simulink model "tracker"  (R2020a)
settings: Solver=VariableStepAuto  StartTime=0.0  StopTime=simulation_time  RelTol=1e-3
values from neighbouring files (symbols this model uses):
  costas_pll_arctan_nstage = 8    [tracker_hw_init.m]
  costas_pll_arctan_point = 16    [tracker_hw_init.m]
  costas_pll_arctan_width = 32    [tracker_hw_init.m]
  DDS_ch_pinc = fc.*(2^(DDS_phase_width)/fs)    [tracker_hw_init.m]
  fs = 120e6    (= 120000000)    [tracker_hw_init.m]
  normalized_EML_power_cordic_nstage = 11    [tracker_hw_init.m]
  normalized_EML_power_cordic_point = 32    [tracker_hw_init.m]
  normalized_EML_power_cordic_width = 32    [tracker_hw_init.m]
  ts = 1/fs    (= 8.33333333333e-09)    [tracker_hw_init.m]
undefined symbols (not defined in the file or in its folder): cacode, i
libraries: xbsIndex_r4 x1873
(part 3 of 14)

== system tracker/CA_code_bank/input_router/address_router1 ==
  ca_select : Inport
  Mux{,1..10} (11 alike) : xbsIndex_r4/Mux  inputs=2  en=off  latency=1  precision=Full  arith_type=Unsigned  n_bits=16  bin_pt=14  quantization=Truncate  overflow=Wrap  dbl_ovrd=off  block_type=mux
  Relational{,1..10} (11 alike) : xbsIndex_r4/Relational  mode=a=b  op_type=Bool  en=off  latency=1  dbl_ovrd=off  block_type=relational
  ca_addr : Outport
  wires:
  [CA_code_addr_ch11] -> Mux10/3
  Mux8/1 -> Mux7/2
  Mux5/1 -> Mux4/2
  [CA_code_select_ch8] -> Relational7/1
  [CA_code_addr_ch9] -> Mux8/3
  [CA_code_select_ch7] -> Relational6/1
  Relational/1 -> Mux/1
  [CA_code_addr_ch1] -> Mux/3
  Mux9/1 -> Mux8/2
  ca_select/1 -> Relational1/2, Relational2/2, Relational3/2, Relational4/2, Relational5/2, Relational6/2, Relational7/2, Relational8/2, Relational9/2, Relational10/2, Relational/2
  Relational9/1 -> Mux9/1
  Mux3/1 -> Mux2/2
  [CA_code_select_ch4] -> Relational3/1
  [CA_code_select_ch3] -> Relational2/1
  Relational8/1 -> Mux8/1
  Relational2/1 -> Mux2/1
  [CA_code_addr_ch5] -> Mux4/3
  [CA_code_select_ch5] -> Relational4/1
  Relational10/1 -> Mux10/1
  Mux2/1 -> Mux1/2
  [CA_code_select_ch2] -> Relational1/1
  Mux4/1 -> Mux3/2
  Relational7/1 -> Mux7/1
  Relational4/1 -> Mux4/1
  [CA_code_select_ch6] -> Relational5/1
  [CA_code_addr_ch6] -> Mux5/3
  [CA_code_addr_ch3] -> Mux2/3
  [CA_code_select_ch1] -> Relational/1
  [CA_code_addr_ch4] -> Mux3/3
  Relational3/1 -> Mux3/1
  [CA_code_select_ch11] -> Relational10/1
  [CA_code_select_ch10] -> Relational9/1
  [CA_code_select_ch9] -> Relational8/1
  Relational5/1 -> Mux5/1
  Mux10/1 -> Mux9/2
  [CA_code_addr_ch10] -> Mux9/3
  Mux7/1 -> Mux6/2
  [CA_code_addr_ch12] -> Mux10/2
  Relational1/1 -> Mux1/1
  [CA_code_addr_ch8] -> Mux7/3
  [CA_code_addr_ch7] -> Mux6/3
  Mux1/1 -> Mux/2
  [CA_code_addr_ch2] -> Mux1/3
  Relational6/1 -> Mux6/1
  Mux6/1 -> Mux5/2
  Mux/1 -> ca_addr/1

== system tracker/CA_code_bank/input_router/address_router10 ==
  ca_select : Inport
  Mux{,1..10} (11 alike) : xbsIndex_r4/Mux  inputs=2  en=off  latency=1  precision=Full  arith_type=Unsigned  n_bits=16  bin_pt=14  quantization=Truncate  overflow=Wrap  dbl_ovrd=off  block_type=mux
  Relational{,1..10} (11 alike) : xbsIndex_r4/Relational  mode=a=b  op_type=Bool  en=off  latency=1  dbl_ovrd=off  block_type=relational
  ca_addr : Outport
  wires:
  [CA_code_addr_ch11] -> Mux10/3
  Mux8/1 -> Mux7/2
  Mux5/1 -> Mux4/2
  [CA_code_select_ch8] -> Relational7/1
  [CA_code_addr_ch9] -> Mux8/3
  [CA_code_select_ch7] -> Relational6/1
  Relational/1 -> Mux/1
  [CA_code_addr_ch1] -> Mux/3
  Mux9/1 -> Mux8/2
  ca_select/1 -> Relational1/2, Relational2/2, Relational3/2, Relational4/2, Relational5/2, Relational6/2, Relational7/2, Relational8/2, Relational9/2, Relational10/2, Relational/2
  Relational9/1 -> Mux9/1
  Mux3/1 -> Mux2/2
  [CA_code_select_ch4] -> Relational3/1
  [CA_code_select_ch3] -> Relational2/1
  Relational8/1 -> Mux8/1
  Relational2/1 -> Mux2/1
  [CA_code_addr_ch5] -> Mux4/3
  [CA_code_select_ch5] -> Relational4/1
  Relational10/1 -> Mux10/1
  Mux2/1 -> Mux1/2
  [CA_code_select_ch2] -> Relational1/1
  Mux4/1 -> Mux3/2
  Relational7/1 -> Mux7/1
  Relational4/1 -> Mux4/1
  [CA_code_select_ch6] -> Relational5/1
  [CA_code_addr_ch6] -> Mux5/3
  [CA_code_addr_ch3] -> Mux2/3
  [CA_code_select_ch1] -> Relational/1
  [CA_code_addr_ch4] -> Mux3/3
  Relational3/1 -> Mux3/1
  [CA_code_select_ch11] -> Relational10/1
  [CA_code_select_ch10] -> Relational9/1
  [CA_code_select_ch9] -> Relational8/1
  Relational5/1 -> Mux5/1
  Mux10/1 -> Mux9/2
  [CA_code_addr_ch10] -> Mux9/3
  Mux7/1 -> Mux6/2
  [CA_code_addr_ch12] -> Mux10/2
  Relational1/1 -> Mux1/1
  [CA_code_addr_ch8] -> Mux7/3
  [CA_code_addr_ch7] -> Mux6/3
  Mux1/1 -> Mux/2
  [CA_code_addr_ch2] -> Mux1/3
  Relational6/1 -> Mux6/1
  Mux6/1 -> Mux5/2
  Mux/1 -> ca_addr/1

== system tracker/CA_code_bank/input_router/address_router11 ==
  ca_select : Inport
  Mux{,1..10} (11 alike) : xbsIndex_r4/Mux  inputs=2  en=off  latency=1  precision=Full  arith_type=Unsigned  n_bits=16  bin_pt=14  quantization=Truncate  overflow=Wrap  dbl_ovrd=off  block_type=mux
  Relational{,1..10} (11 alike) : xbsIndex_r4/Relational  mode=a=b  op_type=Bool  en=off  latency=1  dbl_ovrd=off  block_type=relational
  ca_addr : Outport
  wires:
  Mux/1 -> ca_addr/1
  Mux6/1 -> Mux5/2
  Relational6/1 -> Mux6/1
  [CA_code_addr_ch2] -> Mux1/3
  Mux1/1 -> Mux/2
  [CA_code_addr_ch7] -> Mux6/3
  [CA_code_addr_ch8] -> Mux7/3
  Relational1/1 -> Mux1/1
  [CA_code_addr_ch12] -> Mux10/2
  Mux7/1 -> Mux6/2
  [CA_code_addr_ch10] -> Mux9/3
  Mux10/1 -> Mux9/2
  Relational5/1 -> Mux5/1
  [CA_code_select_ch9] -> Relational8/1
  [CA_code_select_ch10] -> Relational9/1
  [CA_code_select_ch11] -> Relational10/1
  Relational3/1 -> Mux3/1
  [CA_code_addr_ch4] -> Mux3/3
  [CA_code_select_ch1] -> Relational/1
  [CA_code_addr_ch3] -> Mux2/3
  [CA_code_addr_ch6] -> Mux5/3
  [CA_code_select_ch6] -> Relational5/1
  Relational4/1 -> Mux4/1
  Relational7/1 -> Mux7/1
  Mux4/1 -> Mux3/2
  [CA_code_select_ch2] -> Relational1/1
  Mux2/1 -> Mux1/2
  Relational10/1 -> Mux10/1
  [CA_code_select_ch5] -> Relational4/1
  [CA_code_addr_ch5] -> Mux4/3
  Relational2/1 -> Mux2/1
  Relational8/1 -> Mux8/1
  [CA_code_select_ch3] -> Relational2/1
  [CA_code_select_ch4] -> Relational3/1
  Mux3/1 -> Mux2/2
  Relational9/1 -> Mux9/1
  ca_select/1 -> Relational/2, Relational10/2, Relational9/2, Relational8/2, Relational7/2, Relational6/2, Relational5/2, Relational4/2, Relational3/2, Relational2/2, Relational1/2
  Mux9/1 -> Mux8/2
  [CA_code_addr_ch1] -> Mux/3
  Relational/1 -> Mux/1
  [CA_code_select_ch7] -> Relational6/1
  [CA_code_addr_ch9] -> Mux8/3
  [CA_code_select_ch8] -> Relational7/1
  Mux5/1 -> Mux4/2
  Mux8/1 -> Mux7/2
  [CA_code_addr_ch11] -> Mux10/3

== system tracker/CA_code_bank/input_router/address_router12 ==
  ca_select : Inport
  Mux{,1..10} (11 alike) : xbsIndex_r4/Mux  inputs=2  en=off  latency=1  precision=Full  arith_type=Unsigned  n_bits=16  bin_pt=14  quantization=Truncate  overflow=Wrap  dbl_ovrd=off  block_type=mux
  Relational{,1..10} (11 alike) : xbsIndex_r4/Relational  mode=a=b  op_type=Bool  en=off  latency=1  dbl_ovrd=off  block_type=relational
  ca_addr : Outport
  wires:
  [CA_code_addr_ch11] -> Mux10/3
  Mux8/1 -> Mux7/2
  Mux5/1 -> Mux4/2
  [CA_code_select_ch8] -> Relational7/1
  [CA_code_addr_ch9] -> Mux8/3
  [CA_code_select_ch7] -> Relational6/1
  Relational/1 -> Mux/1
  [CA_code_addr_ch1] -> Mux/3
  Mux9/1 -> Mux8/2
  ca_select/1 -> Relational1/2, Relational2/2, Relational3/2, Relational4/2, Relational5/2, Relational6/2, Relational7/2, Relational8/2, Relational9/2, Relational10/2, Relational/2
  Relational9/1 -> Mux9/1
  Mux3/1 -> Mux2/2
  [CA_code_select_ch4] -> Relational3/1
  [CA_code_select_ch3] -> Relational2/1
  Relational8/1 -> Mux8/1
  Relational2/1 -> Mux2/1
  [CA_code_addr_ch5] -> Mux4/3
  [CA_code_select_ch5] -> Relational4/1
  Relational10/1 -> Mux10/1
  Mux2/1 -> Mux1/2
  [CA_code_select_ch2] -> Relational1/1
  Mux4/1 -> Mux3/2
  Relational7/1 -> Mux7/1
  Relational4/1 -> Mux4/1
  [CA_code_select_ch6] -> Relational5/1
  [CA_code_addr_ch6] -> Mux5/3
  [CA_code_addr_ch3] -> Mux2/3
  [CA_code_select_ch1] -> Relational/1
  [CA_code_addr_ch4] -> Mux3/3
  Relational3/1 -> Mux3/1
  [CA_code_select_ch11] -> Relational10/1
  [CA_code_select_ch10] -> Relational9/1
  [CA_code_select_ch9] -> Relational8/1
  Relational5/1 -> Mux5/1
  Mux10/1 -> Mux9/2
  [CA_code_addr_ch10] -> Mux9/3
  Mux7/1 -> Mux6/2
  [CA_code_addr_ch12] -> Mux10/2
  Relational1/1 -> Mux1/1
  [CA_code_addr_ch8] -> Mux7/3
  [CA_code_addr_ch7] -> Mux6/3
  Mux1/1 -> Mux/2
  [CA_code_addr_ch2] -> Mux1/3
  Relational6/1 -> Mux6/1
  Mux6/1 -> Mux5/2
  Mux/1 -> ca_addr/1

== system tracker/CA_code_bank/input_router/address_router13 ==
  ca_select : Inport
  Mux{,1..10} (11 alike) : xbsIndex_r4/Mux  inputs=2  en=off  latency=1  precision=Full  arith_type=Unsigned  n_bits=16  bin_pt=14  quantization=Truncate  overflow=Wrap  dbl_ovrd=off  block_type=mux
  Relational{,1..10} (11 alike) : xbsIndex_r4/Relational  mode=a=b  op_type=Bool  en=off  latency=1  dbl_ovrd=off  block_type=relational
  ca_addr : Outport
  wires:
  Mux/1 -> ca_addr/1
  Mux6/1 -> Mux5/2
  Relational6/1 -> Mux6/1
  [CA_code_addr_ch2] -> Mux1/3
  Mux1/1 -> Mux/2
  [CA_code_addr_ch7] -> Mux6/3
  [CA_code_addr_ch8] -> Mux7/3
  Relational1/1 -> Mux1/1
  [CA_code_addr_ch12] -> Mux10/2
  Mux7/1 -> Mux6/2
  [CA_code_addr_ch10] -> Mux9/3
  Mux10/1 -> Mux9/2
  Relational5/1 -> Mux5/1
  [CA_code_select_ch9] -> Relational8/1
  [CA_code_select_ch10] -> Relational9/1
  [CA_code_select_ch11] -> Relational10/1
  Relational3/1 -> Mux3/1
  [CA_code_addr_ch4] -> Mux3/3
  [CA_code_select_ch1] -> Relational/1
  [CA_code_addr_ch3] -> Mux2/3
  [CA_code_addr_ch6] -> Mux5/3
  [CA_code_select_ch6] -> Relational5/1
  Relational4/1 -> Mux4/1
  Relational7/1 -> Mux7/1
  Mux4/1 -> Mux3/2
  [CA_code_select_ch2] -> Relational1/1
  Mux2/1 -> Mux1/2
  Relational10/1 -> Mux10/1
  [CA_code_select_ch5] -> Relational4/1
  [CA_code_addr_ch5] -> Mux4/3
  Relational2/1 -> Mux2/1
  Relational8/1 -> Mux8/1
  [CA_code_select_ch3] -> Relational2/1
  [CA_code_select_ch4] -> Relational3/1
  Mux3/1 -> Mux2/2
  Relational9/1 -> Mux9/1
  ca_select/1 -> Relational/2, Relational10/2, Relational9/2, Relational8/2, Relational7/2, Relational6/2, Relational5/2, Relational4/2, Relational3/2, Relational2/2, Relational1/2
  Mux9/1 -> Mux8/2
  [CA_code_addr_ch1] -> Mux/3
  Relational/1 -> Mux/1
  [CA_code_select_ch7] -> Relational6/1
  [CA_code_addr_ch9] -> Mux8/3
  [CA_code_select_ch8] -> Relational7/1
  Mux5/1 -> Mux4/2
  Mux8/1 -> Mux7/2
  [CA_code_addr_ch11] -> Mux10/3

== system tracker/CA_code_bank/input_router/address_router14 ==
  ca_select : Inport
  Mux{,1..10} (11 alike) : xbsIndex_r4/Mux  inputs=2  en=off  latency=1  precision=Full  arith_type=Unsigned  n_bits=16  bin_pt=14  quantization=Truncate  overflow=Wrap  dbl_ovrd=off  block_type=mux
  Relational{,1..10} (11 alike) : xbsIndex_r4/Relational  mode=a=b  op_type=Bool  en=off  latency=1  dbl_ovrd=off  block_type=relational
  ca_addr : Outport
  wires:
  Mux/1 -> ca_addr/1
  Mux6/1 -> Mux5/2
  Relational6/1 -> Mux6/1
  [CA_code_addr_ch2] -> Mux1/3
  Mux1/1 -> Mux/2
  [CA_code_addr_ch7] -> Mux6/3
  [CA_code_addr_ch8] -> Mux7/3
  Relational1/1 -> Mux1/1
  [CA_code_addr_ch12] -> Mux10/2
  Mux7/1 -> Mux6/2
  [CA_code_addr_ch10] -> Mux9/3
  Mux10/1 -> Mux9/2
  Relational5/1 -> Mux5/1
  [CA_code_select_ch9] -> Relational8/1
  [CA_code_select_ch10] -> Relational9/1
  [CA_code_select_ch11] -> Relational10/1
  Relational3/1 -> Mux3/1
  [CA_code_addr_ch4] -> Mux3/3
  [CA_code_select_ch1] -> Relational/1
  [CA_code_addr_ch3] -> Mux2/3
  [CA_code_addr_ch6] -> Mux5/3
  [CA_code_select_ch6] -> Relational5/1
  Relational4/1 -> Mux4/1
  Relational7/1 -> Mux7/1
  Mux4/1 -> Mux3/2
  [CA_code_select_ch2] -> Relational1/1
  Mux2/1 -> Mux1/2
  Relational10/1 -> Mux10/1
  [CA_code_select_ch5] -> Relational4/1
  [CA_code_addr_ch5] -> Mux4/3
  Relational2/1 -> Mux2/1
  Relational8/1 -> Mux8/1
  [CA_code_select_ch3] -> Relational2/1
  [CA_code_select_ch4] -> Relational3/1
  Mux3/1 -> Mux2/2
  Relational9/1 -> Mux9/1
  ca_select/1 -> Relational/2, Relational10/2, Relational9/2, Relational8/2, Relational7/2, Relational6/2, Relational5/2, Relational4/2, Relational3/2, Relational2/2, Relational1/2
  Mux9/1 -> Mux8/2
  [CA_code_addr_ch1] -> Mux/3
  Relational/1 -> Mux/1
  [CA_code_select_ch7] -> Relational6/1
  [CA_code_addr_ch9] -> Mux8/3
  [CA_code_select_ch8] -> Relational7/1
  Mux5/1 -> Mux4/2
  Mux8/1 -> Mux7/2
  [CA_code_addr_ch11] -> Mux10/3

== system tracker/CA_code_bank/input_router/address_router15 ==
  ca_select : Inport
  Mux{,1..10} (11 alike) : xbsIndex_r4/Mux  inputs=2  en=off  latency=1  precision=Full  arith_type=Unsigned  n_bits=16  bin_pt=14  quantization=Truncate  overflow=Wrap  dbl_ovrd=off  block_type=mux
  Relational{,1..10} (11 alike) : xbsIndex_r4/Relational  mode=a=b  op_type=Bool  en=off  latency=1  dbl_ovrd=off  block_type=relational
  ca_addr : Outport
  wires:
  [CA_code_addr_ch11] -> Mux10/3
  Mux8/1 -> Mux7/2
  Mux5/1 -> Mux4/2
  [CA_code_select_ch8] -> Relational7/1
  [CA_code_addr_ch9] -> Mux8/3
  [CA_code_select_ch7] -> Relational6/1
  Relational/1 -> Mux/1
  [CA_code_addr_ch1] -> Mux/3
  Mux9/1 -> Mux8/2
  ca_select/1 -> Relational1/2, Relational2/2, Relational3/2, Relational4/2, Relational5/2, Relational6/2, Relational7/2, Relational8/2, Relational9/2, Relational10/2, Relational/2
  Relational9/1 -> Mux9/1
  Mux3/1 -> Mux2/2
  [CA_code_select_ch4] -> Relational3/1
  [CA_code_select_ch3] -> Relational2/1
  Relational8/1 -> Mux8/1
  Relational2/1 -> Mux2/1
  [CA_code_addr_ch5] -> Mux4/3
  [CA_code_select_ch5] -> Relational4/1
  Relational10/1 -> Mux10/1
  Mux2/1 -> Mux1/2
  [CA_code_select_ch2] -> Relational1/1
  Mux4/1 -> Mux3/2
  Relational7/1 -> Mux7/1
  Relational4/1 -> Mux4/1
  [CA_code_select_ch6] -> Relational5/1
  [CA_code_addr_ch6] -> Mux5/3
  [CA_code_addr_ch3] -> Mux2/3
  [CA_code_select_ch1] -> Relational/1
  [CA_code_addr_ch4] -> Mux3/3
  Relational3/1 -> Mux3/1
  [CA_code_select_ch11] -> Relational10/1
  [CA_code_select_ch10] -> Relational9/1
  [CA_code_select_ch9] -> Relational8/1
  Relational5/1 -> Mux5/1
  Mux10/1 -> Mux9/2
  [CA_code_addr_ch10] -> Mux9/3
  Mux7/1 -> Mux6/2
  [CA_code_addr_ch12] -> Mux10/2
  Relational1/1 -> Mux1/1
  [CA_code_addr_ch8] -> Mux7/3
  [CA_code_addr_ch7] -> Mux6/3
  Mux1/1 -> Mux/2
  [CA_code_addr_ch2] -> Mux1/3
  Relational6/1 -> Mux6/1
  Mux6/1 -> Mux5/2
  Mux/1 -> ca_addr/1

== system tracker/CA_code_bank/input_router/address_router16 ==
  ca_select : Inport
  Mux{,1..10} (11 alike) : xbsIndex_r4/Mux  inputs=2  en=off  latency=1  precision=Full  arith_type=Unsigned  n_bits=16  bin_pt=14  quantization=Truncate  overflow=Wrap  dbl_ovrd=off  block_type=mux
  Relational{,1..10} (11 alike) : xbsIndex_r4/Relational  mode=a=b  op_type=Bool  en=off  latency=1  dbl_ovrd=off  block_type=relational
  ca_addr : Outport
  wires:
  Mux/1 -> ca_addr/1
  Mux6/1 -> Mux5/2
  Relational6/1 -> Mux6/1
  [CA_code_addr_ch2] -> Mux1/3
  Mux1/1 -> Mux/2
  [CA_code_addr_ch7] -> Mux6/3
  [CA_code_addr_ch8] -> Mux7/3
  Relational1/1 -> Mux1/1
  [CA_code_addr_ch12] -> Mux10/2
  Mux7/1 -> Mux6/2
  [CA_code_addr_ch10] -> Mux9/3
  Mux10/1 -> Mux9/2
  Relational5/1 -> Mux5/1
  [CA_code_select_ch9] -> Relational8/1
  [CA_code_select_ch10] -> Relational9/1
  [CA_code_select_ch11] -> Relational10/1
  Relational3/1 -> Mux3/1
  [CA_code_addr_ch4] -> Mux3/3
  [CA_code_select_ch1] -> Relational/1
  [CA_code_addr_ch3] -> Mux2/3
  [CA_code_addr_ch6] -> Mux5/3
  [CA_code_select_ch6] -> Relational5/1
  Relational4/1 -> Mux4/1
  Relational7/1 -> Mux7/1
  Mux4/1 -> Mux3/2
  [CA_code_select_ch2] -> Relational1/1
  Mux2/1 -> Mux1/2
  Relational10/1 -> Mux10/1
  [CA_code_select_ch5] -> Relational4/1
  [CA_code_addr_ch5] -> Mux4/3
  Relational2/1 -> Mux2/1
  Relational8/1 -> Mux8/1
  [CA_code_select_ch3] -> Relational2/1
  [CA_code_select_ch4] -> Relational3/1
  Mux3/1 -> Mux2/2
  Relational9/1 -> Mux9/1
  ca_select/1 -> Relational/2, Relational10/2, Relational9/2, Relational8/2, Relational7/2, Relational6/2, Relational5/2, Relational4/2, Relational3/2, Relational2/2, Relational1/2
  Mux9/1 -> Mux8/2
  [CA_code_addr_ch1] -> Mux/3
  Relational/1 -> Mux/1
  [CA_code_select_ch7] -> Relational6/1
  [CA_code_addr_ch9] -> Mux8/3
  [CA_code_select_ch8] -> Relational7/1
  Mux5/1 -> Mux4/2
  Mux8/1 -> Mux7/2
  [CA_code_addr_ch11] -> Mux10/3

== system tracker/CA_code_bank/input_router/address_router17 ==
  ca_select : Inport
  Mux{,1..10} (11 alike) : xbsIndex_r4/Mux  inputs=2  en=off  latency=1  precision=Full  arith_type=Unsigned  n_bits=16  bin_pt=14  quantization=Truncate  overflow=Wrap  dbl_ovrd=off  block_type=mux
  Relational{,1..10} (11 alike) : xbsIndex_r4/Relational  mode=a=b  op_type=Bool  en=off  latency=1  dbl_ovrd=off  block_type=relational
  ca_addr : Outport
  wires:
  [CA_code_addr_ch11] -> Mux10/3
  Mux8/1 -> Mux7/2
  Mux5/1 -> Mux4/2
  [CA_code_select_ch8] -> Relational7/1
  [CA_code_addr_ch9] -> Mux8/3
  [CA_code_select_ch7] -> Relational6/1
  Relational/1 -> Mux/1
  [CA_code_addr_ch1] -> Mux/3
  Mux9/1 -> Mux8/2
  ca_select/1 -> Relational1/2, Relational2/2, Relational3/2, Relational4/2, Relational5/2, Relational6/2, Relational7/2, Relational8/2, Relational9/2, Relational10/2, Relational/2
  Relational9/1 -> Mux9/1
  Mux3/1 -> Mux2/2
  [CA_code_select_ch4] -> Relational3/1
  [CA_code_select_ch3] -> Relational2/1
  Relational8/1 -> Mux8/1
  Relational2/1 -> Mux2/1
  [CA_code_addr_ch5] -> Mux4/3
  [CA_code_select_ch5] -> Relational4/1
  Relational10/1 -> Mux10/1
  Mux2/1 -> Mux1/2
  [CA_code_select_ch2] -> Relational1/1
  Mux4/1 -> Mux3/2
  Relational7/1 -> Mux7/1
  Relational4/1 -> Mux4/1
  [CA_code_select_ch6] -> Relational5/1
  [CA_code_addr_ch6] -> Mux5/3
  [CA_code_addr_ch3] -> Mux2/3
  [CA_code_select_ch1] -> Relational/1
  [CA_code_addr_ch4] -> Mux3/3
  Relational3/1 -> Mux3/1
  [CA_code_select_ch11] -> Relational10/1
  [CA_code_select_ch10] -> Relational9/1
  [CA_code_select_ch9] -> Relational8/1
  Relational5/1 -> Mux5/1
  Mux10/1 -> Mux9/2
  [CA_code_addr_ch10] -> Mux9/3
  Mux7/1 -> Mux6/2
  [CA_code_addr_ch12] -> Mux10/2
  Relational1/1 -> Mux1/1
  [CA_code_addr_ch8] -> Mux7/3
  [CA_code_addr_ch7] -> Mux6/3
  Mux1/1 -> Mux/2
  [CA_code_addr_ch2] -> Mux1/3
  Relational6/1 -> Mux6/1
  Mux6/1 -> Mux5/2
  Mux/1 -> ca_addr/1

== system tracker/CA_code_bank/input_router/address_router18 ==
  ca_select : Inport
  Mux{,1..10} (11 alike) : xbsIndex_r4/Mux  inputs=2  en=off  latency=1  precision=Full  arith_type=Unsigned  n_bits=16  bin_pt=14  quantization=Truncate  overflow=Wrap  dbl_ovrd=off  block_type=mux
  Relational{,1..10} (11 alike) : xbsIndex_r4/Relational  mode=a=b  op_type=Bool  en=off  latency=1  dbl_ovrd=off  block_type=relational
  ca_addr : Outport
  wires:
  Mux/1 -> ca_addr/1
  Mux6/1 -> Mux5/2
  Relational6/1 -> Mux6/1
  [CA_code_addr_ch2] -> Mux1/3
  Mux1/1 -> Mux/2
  [CA_code_addr_ch7] -> Mux6/3
  [CA_code_addr_ch8] -> Mux7/3
  Relational1/1 -> Mux1/1
  [CA_code_addr_ch12] -> Mux10/2
  Mux7/1 -> Mux6/2
  [CA_code_addr_ch10] -> Mux9/3
  Mux10/1 -> Mux9/2
  Relational5/1 -> Mux5/1
  [CA_code_select_ch9] -> Relational8/1
  [CA_code_select_ch10] -> Relational9/1
  [CA_code_select_ch11] -> Relational10/1
  Relational3/1 -> Mux3/1
  [CA_code_addr_ch4] -> Mux3/3
  [CA_code_select_ch1] -> Relational/1
  [CA_code_addr_ch3] -> Mux2/3
  [CA_code_addr_ch6] -> Mux5/3
  [CA_code_select_ch6] -> Relational5/1
  Relational4/1 -> Mux4/1
  Relational7/1 -> Mux7/1
  Mux4/1 -> Mux3/2
  [CA_code_select_ch2] -> Relational1/1
  Mux2/1 -> Mux1/2
  Relational10/1 -> Mux10/1
  [CA_code_select_ch5] -> Relational4/1
  [CA_code_addr_ch5] -> Mux4/3
  Relational2/1 -> Mux2/1
  Relational8/1 -> Mux8/1
  [CA_code_select_ch3] -> Relational2/1
  [CA_code_select_ch4] -> Relational3/1
  Mux3/1 -> Mux2/2
  Relational9/1 -> Mux9/1
  ca_select/1 -> Relational/2, Relational10/2, Relational9/2, Relational8/2, Relational7/2, Relational6/2, Relational5/2, Relational4/2, Relational3/2, Relational2/2, Relational1/2
  Mux9/1 -> Mux8/2
  [CA_code_addr_ch1] -> Mux/3
  Relational/1 -> Mux/1
  [CA_code_select_ch7] -> Relational6/1
  [CA_code_addr_ch9] -> Mux8/3
  [CA_code_select_ch8] -> Relational7/1
  Mux5/1 -> Mux4/2
  Mux8/1 -> Mux7/2
  [CA_code_addr_ch11] -> Mux10/3

== system tracker/CA_code_bank/input_router/address_router19 ==
  ca_select : Inport
  Mux{,1..10} (11 alike) : xbsIndex_r4/Mux  inputs=2  en=off  latency=1  precision=Full  arith_type=Unsigned  n_bits=16  bin_pt=14  quantization=Truncate  overflow=Wrap  dbl_ovrd=off  block_type=mux
  Relational{,1..10} (11 alike) : xbsIndex_r4/Relational  mode=a=b  op_type=Bool  en=off  latency=1  dbl_ovrd=off  block_type=relational
  ca_addr : Outport
  wires:
  [CA_code_addr_ch11] -> Mux10/3
  Mux8/1 -> Mux7/2
  Mux5/1 -> Mux4/2
  [CA_code_select_ch8] -> Relational7/1
  [CA_code_addr_ch9] -> Mux8/3
  [CA_code_select_ch7] -> Relational6/1
  Relational/1 -> Mux/1
  [CA_code_addr_ch1] -> Mux/3
  Mux9/1 -> Mux8/2
  ca_select/1 -> Relational1/2, Relational2/2, Relational3/2, Relational4/2, Relational5/2, Relational6/2, Relational7/2, Relational8/2, Relational9/2, Relational10/2, Relational/2
  Relational9/1 -> Mux9/1
  Mux3/1 -> Mux2/2
  [CA_code_select_ch4] -> Relational3/1
  [CA_code_select_ch3] -> Relational2/1
  Relational8/1 -> Mux8/1
  Relational2/1 -> Mux2/1
  [CA_code_addr_ch5] -> Mux4/3
  [CA_code_select_ch5] -> Relational4/1
  Relational10/1 -> Mux10/1
  Mux2/1 -> Mux1/2
  [CA_code_select_ch2] -> Relational1/1
  Mux4/1 -> Mux3/2
  Relational7/1 -> Mux7/1
  Relational4/1 -> Mux4/1
  [CA_code_select_ch6] -> Relational5/1
  [CA_code_addr_ch6] -> Mux5/3
  [CA_code_addr_ch3] -> Mux2/3
  [CA_code_select_ch1] -> Relational/1
  [CA_code_addr_ch4] -> Mux3/3
  Relational3/1 -> Mux3/1
  [CA_code_select_ch11] -> Relational10/1
  [CA_code_select_ch10] -> Relational9/1
  [CA_code_select_ch9] -> Relational8/1
  Relational5/1 -> Mux5/1
  Mux10/1 -> Mux9/2
  [CA_code_addr_ch10] -> Mux9/3
  Mux7/1 -> Mux6/2
  [CA_code_addr_ch12] -> Mux10/2
  Relational1/1 -> Mux1/1
  [CA_code_addr_ch8] -> Mux7/3
  [CA_code_addr_ch7] -> Mux6/3
  Mux1/1 -> Mux/2
  [CA_code_addr_ch2] -> Mux1/3
  Relational6/1 -> Mux6/1
  Mux6/1 -> Mux5/2
  Mux/1 -> ca_addr/1

== system tracker/CA_code_bank/input_router/address_router2 ==
  ca_select : Inport
  Mux{,1..10} (11 alike) : xbsIndex_r4/Mux  inputs=2  en=off  latency=1  precision=Full  arith_type=Unsigned  n_bits=16  bin_pt=14  quantization=Truncate  overflow=Wrap  dbl_ovrd=off  block_type=mux
  Relational{,1..10} (11 alike) : xbsIndex_r4/Relational  mode=a=b  op_type=Bool  en=off  latency=1  dbl_ovrd=off  block_type=relational
  ca_addr : Outport
  wires:
  Mux/1 -> ca_addr/1
  Mux6/1 -> Mux5/2
  Relational6/1 -> Mux6/1
  [CA_code_addr_ch2] -> Mux1/3
  Mux1/1 -> Mux/2
  [CA_code_addr_ch7] -> Mux6/3
  [CA_code_addr_ch8] -> Mux7/3
  Relational1/1 -> Mux1/1
  [CA_code_addr_ch12] -> Mux10/2
  Mux7/1 -> Mux6/2
  [CA_code_addr_ch10] -> Mux9/3
  Mux10/1 -> Mux9/2
  Relational5/1 -> Mux5/1
  [CA_code_select_ch9] -> Relational8/1
  [CA_code_select_ch10] -> Relational9/1
  [CA_code_select_ch11] -> Relational10/1
  Relational3/1 -> Mux3/1
  [CA_code_addr_ch4] -> Mux3/3
  [CA_code_select_ch1] -> Relational/1
  [CA_code_addr_ch3] -> Mux2/3
  [CA_code_addr_ch6] -> Mux5/3
  [CA_code_select_ch6] -> Relational5/1
  Relational4/1 -> Mux4/1
  Relational7/1 -> Mux7/1
  Mux4/1 -> Mux3/2
  [CA_code_select_ch2] -> Relational1/1
  Mux2/1 -> Mux1/2
  Relational10/1 -> Mux10/1
  [CA_code_select_ch5] -> Relational4/1
  [CA_code_addr_ch5] -> Mux4/3
  Relational2/1 -> Mux2/1
  Relational8/1 -> Mux8/1
  [CA_code_select_ch3] -> Relational2/1
  [CA_code_select_ch4] -> Relational3/1
  Mux3/1 -> Mux2/2
  Relational9/1 -> Mux9/1
  ca_select/1 -> Relational/2, Relational10/2, Relational9/2, Relational8/2, Relational7/2, Relational6/2, Relational5/2, Relational4/2, Relational3/2, Relational2/2, Relational1/2
  Mux9/1 -> Mux8/2
  [CA_code_addr_ch1] -> Mux/3
  Relational/1 -> Mux/1
  [CA_code_select_ch7] -> Relational6/1
  [CA_code_addr_ch9] -> Mux8/3
  [CA_code_select_ch8] -> Relational7/1
  Mux5/1 -> Mux4/2
  Mux8/1 -> Mux7/2
  [CA_code_addr_ch11] -> Mux10/3

== system tracker/CA_code_bank/input_router/address_router20 ==
  ca_select : Inport
  Mux{,1..10} (11 alike) : xbsIndex_r4/Mux  inputs=2  en=off  latency=1  precision=Full  arith_type=Unsigned  n_bits=16  bin_pt=14  quantization=Truncate  overflow=Wrap  dbl_ovrd=off  block_type=mux
  Relational{,1..10} (11 alike) : xbsIndex_r4/Relational  mode=a=b  op_type=Bool  en=off  latency=1  dbl_ovrd=off  block_type=relational
  ca_addr : Outport
  wires:
  Mux/1 -> ca_addr/1
  Mux6/1 -> Mux5/2
  Relational6/1 -> Mux6/1
  [CA_code_addr_ch2] -> Mux1/3
  Mux1/1 -> Mux/2
  [CA_code_addr_ch7] -> Mux6/3
  [CA_code_addr_ch8] -> Mux7/3
  Relational1/1 -> Mux1/1
  [CA_code_addr_ch12] -> Mux10/2
  Mux7/1 -> Mux6/2
  [CA_code_addr_ch10] -> Mux9/3
  Mux10/1 -> Mux9/2
  Relational5/1 -> Mux5/1
  [CA_code_select_ch9] -> Relational8/1
  [CA_code_select_ch10] -> Relational9/1
  [CA_code_select_ch11] -> Relational10/1
  Relational3/1 -> Mux3/1
  [CA_code_addr_ch4] -> Mux3/3
  [CA_code_select_ch1] -> Relational/1
  [CA_code_addr_ch3] -> Mux2/3
  [CA_code_addr_ch6] -> Mux5/3
  [CA_code_select_ch6] -> Relational5/1
  Relational4/1 -> Mux4/1
  Relational7/1 -> Mux7/1
  Mux4/1 -> Mux3/2
  [CA_code_select_ch2] -> Relational1/1
  Mux2/1 -> Mux1/2
  Relational10/1 -> Mux10/1
  [CA_code_select_ch5] -> Relational4/1
  [CA_code_addr_ch5] -> Mux4/3
  Relational2/1 -> Mux2/1
  Relational8/1 -> Mux8/1
  [CA_code_select_ch3] -> Relational2/1
  [CA_code_select_ch4] -> Relational3/1
  Mux3/1 -> Mux2/2
  Relational9/1 -> Mux9/1
  ca_select/1 -> Relational/2, Relational10/2, Relational9/2, Relational8/2, Relational7/2, Relational6/2, Relational5/2, Relational4/2, Relational3/2, Relational2/2, Relational1/2
  Mux9/1 -> Mux8/2
  [CA_code_addr_ch1] -> Mux/3
  Relational/1 -> Mux/1
  [CA_code_select_ch7] -> Relational6/1
  [CA_code_addr_ch9] -> Mux8/3
  [CA_code_select_ch8] -> Relational7/1
  Mux5/1 -> Mux4/2
  Mux8/1 -> Mux7/2
  [CA_code_addr_ch11] -> Mux10/3

== system tracker/CA_code_bank/input_router/address_router21 ==
  ca_select : Inport
  Mux{,1..10} (11 alike) : xbsIndex_r4/Mux  inputs=2  en=off  latency=1  precision=Full  arith_type=Unsigned  n_bits=16  bin_pt=14  quantization=Truncate  overflow=Wrap  dbl_ovrd=off  block_type=mux
  Relational{,1..10} (11 alike) : xbsIndex_r4/Relational  mode=a=b  op_type=Bool  en=off  latency=1  dbl_ovrd=off  block_type=relational
  ca_addr : Outport
  wires:
  [CA_code_addr_ch11] -> Mux10/3
  Mux8/1 -> Mux7/2
  Mux5/1 -> Mux4/2
  [CA_code_select_ch8] -> Relational7/1
  [CA_code_addr_ch9] -> Mux8/3
  [CA_code_select_ch7] -> Relational6/1
  Relational/1 -> Mux/1
  [CA_code_addr_ch1] -> Mux/3
  Mux9/1 -> Mux8/2
  ca_select/1 -> Relational1/2, Relational2/2, Relational3/2, Relational4/2, Relational5/2, Relational6/2, Relational7/2, Relational8/2, Relational9/2, Relational10/2, Relational/2
  Relational9/1 -> Mux9/1
  Mux3/1 -> Mux2/2
  [CA_code_select_ch4] -> Relational3/1
  [CA_code_select_ch3] -> Relational2/1
  Relational8/1 -> Mux8/1
  Relational2/1 -> Mux2/1
  [CA_code_addr_ch5] -> Mux4/3
  [CA_code_select_ch5] -> Relational4/1
  Relational10/1 -> Mux10/1
  Mux2/1 -> Mux1/2
  [CA_code_select_ch2] -> Relational1/1
  Mux4/1 -> Mux3/2
  Relational7/1 -> Mux7/1
  Relational4/1 -> Mux4/1
  [CA_code_select_ch6] -> Relational5/1
  [CA_code_addr_ch6] -> Mux5/3
  [CA_code_addr_ch3] -> Mux2/3
  [CA_code_select_ch1] -> Relational/1
  [CA_code_addr_ch4] -> Mux3/3
  Relational3/1 -> Mux3/1
  [CA_code_select_ch11] -> Relational10/1
  [CA_code_select_ch10] -> Relational9/1
  [CA_code_select_ch9] -> Relational8/1
  Relational5/1 -> Mux5/1
  Mux10/1 -> Mux9/2
  [CA_code_addr_ch10] -> Mux9/3
  Mux7/1 -> Mux6/2
  [CA_code_addr_ch12] -> Mux10/2
  Relational1/1 -> Mux1/1
  [CA_code_addr_ch8] -> Mux7/3
  [CA_code_addr_ch7] -> Mux6/3
  Mux1/1 -> Mux/2
  [CA_code_addr_ch2] -> Mux1/3
  Relational6/1 -> Mux6/1
  Mux6/1 -> Mux5/2
  Mux/1 -> ca_addr/1

== system tracker/CA_code_bank/input_router/address_router22 ==
  ca_select : Inport
  Mux{,1..10} (11 alike) : xbsIndex_r4/Mux  inputs=2  en=off  latency=1  precision=Full  arith_type=Unsigned  n_bits=16  bin_pt=14  quantization=Truncate  overflow=Wrap  dbl_ovrd=off  block_type=mux
  Relational{,1..10} (11 alike) : xbsIndex_r4/Relational  mode=a=b  op_type=Bool  en=off  latency=1  dbl_ovrd=off  block_type=relational
  ca_addr : Outport
  wires:
  [CA_code_addr_ch11] -> Mux10/3
  Mux8/1 -> Mux7/2
  Mux5/1 -> Mux4/2
  [CA_code_select_ch8] -> Relational7/1
  [CA_code_addr_ch9] -> Mux8/3
  [CA_code_select_ch7] -> Relational6/1
  Relational/1 -> Mux/1
  [CA_code_addr_ch1] -> Mux/3
  Mux9/1 -> Mux8/2
  ca_select/1 -> Relational1/2, Relational2/2, Relational3/2, Relational4/2, Relational5/2, Relational6/2, Relational7/2, Relational8/2, Relational9/2, Relational10/2, Relational/2
  Relational9/1 -> Mux9/1
  Mux3/1 -> Mux2/2
  [CA_code_select_ch4] -> Relational3/1
  [CA_code_select_ch3] -> Relational2/1
  Relational8/1 -> Mux8/1
  Relational2/1 -> Mux2/1
  [CA_code_addr_ch5] -> Mux4/3
  [CA_code_select_ch5] -> Relational4/1
  Relational10/1 -> Mux10/1
  Mux2/1 -> Mux1/2
  [CA_code_select_ch2] -> Relational1/1
  Mux4/1 -> Mux3/2
  Relational7/1 -> Mux7/1
  Relational4/1 -> Mux4/1
  [CA_code_select_ch6] -> Relational5/1
  [CA_code_addr_ch6] -> Mux5/3
  [CA_code_addr_ch3] -> Mux2/3
  [CA_code_select_ch1] -> Relational/1
  [CA_code_addr_ch4] -> Mux3/3
  Relational3/1 -> Mux3/1
  [CA_code_select_ch11] -> Relational10/1
  [CA_code_select_ch10] -> Relational9/1
  [CA_code_select_ch9] -> Relational8/1
  Relational5/1 -> Mux5/1
  Mux10/1 -> Mux9/2
  [CA_code_addr_ch10] -> Mux9/3
  Mux7/1 -> Mux6/2
  [CA_code_addr_ch12] -> Mux10/2
  Relational1/1 -> Mux1/1
  [CA_code_addr_ch8] -> Mux7/3
  [CA_code_addr_ch7] -> Mux6/3
  Mux1/1 -> Mux/2
  [CA_code_addr_ch2] -> Mux1/3
  Relational6/1 -> Mux6/1
  Mux6/1 -> Mux5/2
  Mux/1 -> ca_addr/1

== system tracker/CA_code_bank/input_router/address_router23 ==
  ca_select : Inport
  Mux{,1..10} (11 alike) : xbsIndex_r4/Mux  inputs=2  en=off  latency=1  precision=Full  arith_type=Unsigned  n_bits=16  bin_pt=14  quantization=Truncate  overflow=Wrap  dbl_ovrd=off  block_type=mux
  Relational{,1..10} (11 alike) : xbsIndex_r4/Relational  mode=a=b  op_type=Bool  en=off  latency=1  dbl_ovrd=off  block_type=relational
  ca_addr : Outport
  wires:
  Mux/1 -> ca_addr/1
  Mux6/1 -> Mux5/2
  Relational6/1 -> Mux6/1
  [CA_code_addr_ch2] -> Mux1/3
  Mux1/1 -> Mux/2
  [CA_code_addr_ch7] -> Mux6/3
  [CA_code_addr_ch8] -> Mux7/3
  Relational1/1 -> Mux1/1
  [CA_code_addr_ch12] -> Mux10/2
  Mux7/1 -> Mux6/2
  [CA_code_addr_ch10] -> Mux9/3
  Mux10/1 -> Mux9/2
  Relational5/1 -> Mux5/1
  [CA_code_select_ch9] -> Relational8/1
  [CA_code_select_ch10] -> Relational9/1
  [CA_code_select_ch11] -> Relational10/1
  Relational3/1 -> Mux3/1
  [CA_code_addr_ch4] -> Mux3/3
  [CA_code_select_ch1] -> Relational/1
  [CA_code_addr_ch3] -> Mux2/3
  [CA_code_addr_ch6] -> Mux5/3
  [CA_code_select_ch6] -> Relational5/1
  Relational4/1 -> Mux4/1
  Relational7/1 -> Mux7/1
  Mux4/1 -> Mux3/2
  [CA_code_select_ch2] -> Relational1/1
  Mux2/1 -> Mux1/2
  Relational10/1 -> Mux10/1
  [CA_code_select_ch5] -> Relational4/1
  [CA_code_addr_ch5] -> Mux4/3
  Relational2/1 -> Mux2/1
  Relational8/1 -> Mux8/1
  [CA_code_select_ch3] -> Relational2/1
  [CA_code_select_ch4] -> Relational3/1
  Mux3/1 -> Mux2/2
  Relational9/1 -> Mux9/1
  ca_select/1 -> Relational/2, Relational10/2, Relational9/2, Relational8/2, Relational7/2, Relational6/2, Relational5/2, Relational4/2, Relational3/2, Relational2/2, Relational1/2
  Mux9/1 -> Mux8/2
  [CA_code_addr_ch1] -> Mux/3
  Relational/1 -> Mux/1
  [CA_code_select_ch7] -> Relational6/1
  [CA_code_addr_ch9] -> Mux8/3
  [CA_code_select_ch8] -> Relational7/1
  Mux5/1 -> Mux4/2
  Mux8/1 -> Mux7/2
  [CA_code_addr_ch11] -> Mux10/3

== system tracker/CA_code_bank/input_router/address_router24 ==
  ca_select : Inport
  Mux{,1..10} (11 alike) : xbsIndex_r4/Mux  inputs=2  en=off  latency=1  precision=Full  arith_type=Unsigned  n_bits=16  bin_pt=14  quantization=Truncate  overflow=Wrap  dbl_ovrd=off  block_type=mux
  Relational{,1..10} (11 alike) : xbsIndex_r4/Relational  mode=a=b  op_type=Bool  en=off  latency=1  dbl_ovrd=off  block_type=relational
  ca_addr : Outport
  wires:
  [CA_code_addr_ch11] -> Mux10/3
  Mux8/1 -> Mux7/2
  Mux5/1 -> Mux4/2
  [CA_code_select_ch8] -> Relational7/1
  [CA_code_addr_ch9] -> Mux8/3
  [CA_code_select_ch7] -> Relational6/1
  Relational/1 -> Mux/1
  [CA_code_addr_ch1] -> Mux/3
  Mux9/1 -> Mux8/2
  ca_select/1 -> Relational1/2, Relational2/2, Relational3/2, Relational4/2, Relational5/2, Relational6/2, Relational7/2, Relational8/2, Relational9/2, Relational10/2, Relational/2
  Relational9/1 -> Mux9/1
  Mux3/1 -> Mux2/2
  [CA_code_select_ch4] -> Relational3/1
  [CA_code_select_ch3] -> Relational2/1
  Relational8/1 -> Mux8/1
  Relational2/1 -> Mux2/1
  [CA_code_addr_ch5] -> Mux4/3
  [CA_code_select_ch5] -> Relational4/1
  Relational10/1 -> Mux10/1
  Mux2/1 -> Mux1/2
  [CA_code_select_ch2] -> Relational1/1
  Mux4/1 -> Mux3/2
  Relational7/1 -> Mux7/1
  Relational4/1 -> Mux4/1
  [CA_code_select_ch6] -> Relational5/1
  [CA_code_addr_ch6] -> Mux5/3
  [CA_code_addr_ch3] -> Mux2/3
  [CA_code_select_ch1] -> Relational/1
  [CA_code_addr_ch4] -> Mux3/3
  Relational3/1 -> Mux3/1
  [CA_code_select_ch11] -> Relational10/1
  [CA_code_select_ch10] -> Relational9/1
  [CA_code_select_ch9] -> Relational8/1
  Relational5/1 -> Mux5/1
  Mux10/1 -> Mux9/2
  [CA_code_addr_ch10] -> Mux9/3
  Mux7/1 -> Mux6/2
  [CA_code_addr_ch12] -> Mux10/2
  Relational1/1 -> Mux1/1
  [CA_code_addr_ch8] -> Mux7/3
  [CA_code_addr_ch7] -> Mux6/3
  Mux1/1 -> Mux/2
  [CA_code_addr_ch2] -> Mux1/3
  Relational6/1 -> Mux6/1
  Mux6/1 -> Mux5/2
  Mux/1 -> ca_addr/1

== system tracker/CA_code_bank/input_router/address_router25 ==
  ca_select : Inport
  Mux{,1..10} (11 alike) : xbsIndex_r4/Mux  inputs=2  en=off  latency=1  precision=Full  arith_type=Unsigned  n_bits=16  bin_pt=14  quantization=Truncate  overflow=Wrap  dbl_ovrd=off  block_type=mux
  Relational{,1..10} (11 alike) : xbsIndex_r4/Relational  mode=a=b  op_type=Bool  en=off  latency=1  dbl_ovrd=off  block_type=relational
  ca_addr : Outport
  wires:
  [CA_code_addr_ch11] -> Mux10/3
  Mux8/1 -> Mux7/2
  Mux5/1 -> Mux4/2
  [CA_code_select_ch8] -> Relational7/1
  [CA_code_addr_ch9] -> Mux8/3
  [CA_code_select_ch7] -> Relational6/1
  Relational/1 -> Mux/1
  [CA_code_addr_ch1] -> Mux/3
  Mux9/1 -> Mux8/2
  ca_select/1 -> Relational1/2, Relational2/2, Relational3/2, Relational4/2, Relational5/2, Relational6/2, Relational7/2, Relational8/2, Relational9/2, Relational10/2, Relational/2
  Relational9/1 -> Mux9/1
  Mux3/1 -> Mux2/2
  [CA_code_select_ch4] -> Relational3/1
  [CA_code_select_ch3] -> Relational2/1
  Relational8/1 -> Mux8/1
  Relational2/1 -> Mux2/1
  [CA_code_addr_ch5] -> Mux4/3
  [CA_code_select_ch5] -> Relational4/1
  Relational10/1 -> Mux10/1
  Mux2/1 -> Mux1/2
  [CA_code_select_ch2] -> Relational1/1
  Mux4/1 -> Mux3/2
  Relational7/1 -> Mux7/1
  Relational4/1 -> Mux4/1
  [CA_code_select_ch6] -> Relational5/1
  [CA_code_addr_ch6] -> Mux5/3
  [CA_code_addr_ch3] -> Mux2/3
  [CA_code_select_ch1] -> Relational/1
  [CA_code_addr_ch4] -> Mux3/3
  Relational3/1 -> Mux3/1
  [CA_code_select_ch11] -> Relational10/1
  [CA_code_select_ch10] -> Relational9/1
  [CA_code_select_ch9] -> Relational8/1
  Relational5/1 -> Mux5/1
  Mux10/1 -> Mux9/2
  [CA_code_addr_ch10] -> Mux9/3
  Mux7/1 -> Mux6/2
  [CA_code_addr_ch12] -> Mux10/2
  Relational1/1 -> Mux1/1
  [CA_code_addr_ch8] -> Mux7/3
  [CA_code_addr_ch7] -> Mux6/3
  Mux1/1 -> Mux/2
  [CA_code_addr_ch2] -> Mux1/3
  Relational6/1 -> Mux6/1
  Mux6/1 -> Mux5/2
  Mux/1 -> ca_addr/1

== system tracker/CA_code_bank/input_router/address_router26 ==
  ca_select : Inport
  Mux{,1..10} (11 alike) : xbsIndex_r4/Mux  inputs=2  en=off  latency=1  precision=Full  arith_type=Unsigned  n_bits=16  bin_pt=14  quantization=Truncate  overflow=Wrap  dbl_ovrd=off  block_type=mux
  Relational{,1..10} (11 alike) : xbsIndex_r4/Relational  mode=a=b  op_type=Bool  en=off  latency=1  dbl_ovrd=off  block_type=relational
  ca_addr : Outport
  wires:
  [CA_code_addr_ch11] -> Mux10/3
  Mux8/1 -> Mux7/2
  Mux5/1 -> Mux4/2
  [CA_code_select_ch8] -> Relational7/1
  [CA_code_addr_ch9] -> Mux8/3
  [CA_code_select_ch7] -> Relational6/1
  Relational/1 -> Mux/1
  [CA_code_addr_ch1] -> Mux/3
  Mux9/1 -> Mux8/2
  ca_select/1 -> Relational1/2, Relational2/2, Relational3/2, Relational4/2, Relational5/2, Relational6/2, Relational7/2, Relational8/2, Relational9/2, Relational10/2, Relational/2
  Relational9/1 -> Mux9/1
  Mux3/1 -> Mux2/2
  [CA_code_select_ch4] -> Relational3/1
  [CA_code_select_ch3] -> Relational2/1
  Relational8/1 -> Mux8/1
  Relational2/1 -> Mux2/1
  [CA_code_addr_ch5] -> Mux4/3
  [CA_code_select_ch5] -> Relational4/1
  Relational10/1 -> Mux10/1
  Mux2/1 -> Mux1/2
  [CA_code_select_ch2] -> Relational1/1
  Mux4/1 -> Mux3/2
  Relational7/1 -> Mux7/1
  Relational4/1 -> Mux4/1
  [CA_code_select_ch6] -> Relational5/1
  [CA_code_addr_ch6] -> Mux5/3
  [CA_code_addr_ch3] -> Mux2/3
  [CA_code_select_ch1] -> Relational/1
  [CA_code_addr_ch4] -> Mux3/3
  Relational3/1 -> Mux3/1
  [CA_code_select_ch11] -> Relational10/1
  [CA_code_select_ch10] -> Relational9/1
  [CA_code_select_ch9] -> Relational8/1
  Relational5/1 -> Mux5/1
  Mux10/1 -> Mux9/2
  [CA_code_addr_ch10] -> Mux9/3
  Mux7/1 -> Mux6/2
  [CA_code_addr_ch12] -> Mux10/2
  Relational1/1 -> Mux1/1
  [CA_code_addr_ch8] -> Mux7/3
  [CA_code_addr_ch7] -> Mux6/3
  Mux1/1 -> Mux/2
  [CA_code_addr_ch2] -> Mux1/3
  Relational6/1 -> Mux6/1
  Mux6/1 -> Mux5/2
  Mux/1 -> ca_addr/1

== system tracker/CA_code_bank/input_router/address_router27 ==
  ca_select : Inport
  Mux{,1..10} (11 alike) : xbsIndex_r4/Mux  inputs=2  en=off  latency=1  precision=Full  arith_type=Unsigned  n_bits=16  bin_pt=14  quantization=Truncate  overflow=Wrap  dbl_ovrd=off  block_type=mux
  Relational{,1..10} (11 alike) : xbsIndex_r4/Relational  mode=a=b  op_type=Bool  en=off  latency=1  dbl_ovrd=off  block_type=relational
  ca_addr : Outport
  wires:
  Mux/1 -> ca_addr/1
  Mux6/1 -> Mux5/2
  Relational6/1 -> Mux6/1
  [CA_code_addr_ch2] -> Mux1/3
  Mux1/1 -> Mux/2
  [CA_code_addr_ch7] -> Mux6/3
  [CA_code_addr_ch8] -> Mux7/3
  Relational1/1 -> Mux1/1
  [CA_code_addr_ch12] -> Mux10/2
  Mux7/1 -> Mux6/2
  [CA_code_addr_ch10] -> Mux9/3
  Mux10/1 -> Mux9/2
  Relational5/1 -> Mux5/1
  [CA_code_select_ch9] -> Relational8/1
  [CA_code_select_ch10] -> Relational9/1
  [CA_code_select_ch11] -> Relational10/1
  Relational3/1 -> Mux3/1
  [CA_code_addr_ch4] -> Mux3/3
  [CA_code_select_ch1] -> Relational/1
  [CA_code_addr_ch3] -> Mux2/3
  [CA_code_addr_ch6] -> Mux5/3
  [CA_code_select_ch6] -> Relational5/1
  Relational4/1 -> Mux4/1
  Relational7/1 -> Mux7/1
  Mux4/1 -> Mux3/2
  [CA_code_select_ch2] -> Relational1/1
  Mux2/1 -> Mux1/2
  Relational10/1 -> Mux10/1
  [CA_code_select_ch5] -> Relational4/1
  [CA_code_addr_ch5] -> Mux4/3
  Relational2/1 -> Mux2/1
  Relational8/1 -> Mux8/1
  [CA_code_select_ch3] -> Relational2/1
  [CA_code_select_ch4] -> Relational3/1
  Mux3/1 -> Mux2/2
  Relational9/1 -> Mux9/1
  ca_select/1 -> Relational/2, Relational10/2, Relational9/2, Relational8/2, Relational7/2, Relational6/2, Relational5/2, Relational4/2, Relational3/2, Relational2/2, Relational1/2
  Mux9/1 -> Mux8/2
  [CA_code_addr_ch1] -> Mux/3
  Relational/1 -> Mux/1
  [CA_code_select_ch7] -> Relational6/1
  [CA_code_addr_ch9] -> Mux8/3
  [CA_code_select_ch8] -> Relational7/1
  Mux5/1 -> Mux4/2
  Mux8/1 -> Mux7/2
  [CA_code_addr_ch11] -> Mux10/3

== system tracker/CA_code_bank/input_router/address_router28 ==
  ca_select : Inport
  Mux{,1..10} (11 alike) : xbsIndex_r4/Mux  inputs=2  en=off  latency=1  precision=Full  arith_type=Unsigned  n_bits=16  bin_pt=14  quantization=Truncate  overflow=Wrap  dbl_ovrd=off  block_type=mux
  Relational{,1..10} (11 alike) : xbsIndex_r4/Relational  mode=a=b  op_type=Bool  en=off  latency=1  dbl_ovrd=off  block_type=relational
  ca_addr : Outport
  wires:
  [CA_code_addr_ch11] -> Mux10/3
  Mux8/1 -> Mux7/2
  Mux5/1 -> Mux4/2
  [CA_code_select_ch8] -> Relational7/1
  [CA_code_addr_ch9] -> Mux8/3
  [CA_code_select_ch7] -> Relational6/1
  Relational/1 -> Mux/1
  [CA_code_addr_ch1] -> Mux/3
  Mux9/1 -> Mux8/2
  ca_select/1 -> Relational1/2, Relational2/2, Relational3/2, Relational4/2, Relational5/2, Relational6/2, Relational7/2, Relational8/2, Relational9/2, Relational10/2, Relational/2
  Relational9/1 -> Mux9/1
  Mux3/1 -> Mux2/2
  [CA_code_select_ch4] -> Relational3/1
  [CA_code_select_ch3] -> Relational2/1
  Relational8/1 -> Mux8/1
  Relational2/1 -> Mux2/1
  [CA_code_addr_ch5] -> Mux4/3
  [CA_code_select_ch5] -> Relational4/1
  Relational10/1 -> Mux10/1
  Mux2/1 -> Mux1/2
  [CA_code_select_ch2] -> Relational1/1
  Mux4/1 -> Mux3/2
  Relational7/1 -> Mux7/1
  Relational4/1 -> Mux4/1
  [CA_code_select_ch6] -> Relational5/1
  [CA_code_addr_ch6] -> Mux5/3
  [CA_code_addr_ch3] -> Mux2/3
  [CA_code_select_ch1] -> Relational/1
  [CA_code_addr_ch4] -> Mux3/3
  Relational3/1 -> Mux3/1
  [CA_code_select_ch11] -> Relational10/1
  [CA_code_select_ch10] -> Relational9/1
  [CA_code_select_ch9] -> Relational8/1
  Relational5/1 -> Mux5/1
  Mux10/1 -> Mux9/2
  [CA_code_addr_ch10] -> Mux9/3
  Mux7/1 -> Mux6/2
  [CA_code_addr_ch12] -> Mux10/2
  Relational1/1 -> Mux1/1
  [CA_code_addr_ch8] -> Mux7/3
  [CA_code_addr_ch7] -> Mux6/3
  Mux1/1 -> Mux/2
  [CA_code_addr_ch2] -> Mux1/3
  Relational6/1 -> Mux6/1
  Mux6/1 -> Mux5/2
  Mux/1 -> ca_addr/1

== system tracker/CA_code_bank/input_router/address_router29 ==
  ca_select : Inport
  Mux{,1..10} (11 alike) : xbsIndex_r4/Mux  inputs=2  en=off  latency=1  precision=Full  arith_type=Unsigned  n_bits=16  bin_pt=14  quantization=Truncate  overflow=Wrap  dbl_ovrd=off  block_type=mux
  Relational{,1..10} (11 alike) : xbsIndex_r4/Relational  mode=a=b  op_type=Bool  en=off  latency=1  dbl_ovrd=off  block_type=relational
  ca_addr : Outport
  wires:
  Mux/1 -> ca_addr/1
  Mux6/1 -> Mux5/2
  Relational6/1 -> Mux6/1
  [CA_code_addr_ch2] -> Mux1/3
  Mux1/1 -> Mux/2
  [CA_code_addr_ch7] -> Mux6/3
  [CA_code_addr_ch8] -> Mux7/3
  Relational1/1 -> Mux1/1
  [CA_code_addr_ch12] -> Mux10/2
  Mux7/1 -> Mux6/2
  [CA_code_addr_ch10] -> Mux9/3
  Mux10/1 -> Mux9/2
  Relational5/1 -> Mux5/1
  [CA_code_select_ch9] -> Relational8/1
  [CA_code_select_ch10] -> Relational9/1
  [CA_code_select_ch11] -> Relational10/1
  Relational3/1 -> Mux3/1
  [CA_code_addr_ch4] -> Mux3/3
  [CA_code_select_ch1] -> Relational/1
  [CA_code_addr_ch3] -> Mux2/3
  [CA_code_addr_ch6] -> Mux5/3
  [CA_code_select_ch6] -> Relational5/1
  Relational4/1 -> Mux4/1
  Relational7/1 -> Mux7/1
  Mux4/1 -> Mux3/2
  [CA_code_select_ch2] -> Relational1/1
  Mux2/1 -> Mux1/2
  Relational10/1 -> Mux10/1
  [CA_code_select_ch5] -> Relational4/1
  [CA_code_addr_ch5] -> Mux4/3
  Relational2/1 -> Mux2/1
  Relational8/1 -> Mux8/1
  [CA_code_select_ch3] -> Relational2/1
  [CA_code_select_ch4] -> Relational3/1
  Mux3/1 -> Mux2/2
  Relational9/1 -> Mux9/1
  ca_select/1 -> Relational/2, Relational10/2, Relational9/2, Relational8/2, Relational7/2, Relational6/2, Relational5/2, Relational4/2, Relational3/2, Relational2/2, Relational1/2
  Mux9/1 -> Mux8/2
  [CA_code_addr_ch1] -> Mux/3
  Relational/1 -> Mux/1
  [CA_code_select_ch7] -> Relational6/1
  [CA_code_addr_ch9] -> Mux8/3
  [CA_code_select_ch8] -> Relational7/1
  Mux5/1 -> Mux4/2
  Mux8/1 -> Mux7/2
  [CA_code_addr_ch11] -> Mux10/3

== system tracker/CA_code_bank/input_router/address_router3 ==
  ca_select : Inport
  Mux{,1..10} (11 alike) : xbsIndex_r4/Mux  inputs=2  en=off  latency=1  precision=Full  arith_type=Unsigned  n_bits=16  bin_pt=14  quantization=Truncate  overflow=Wrap  dbl_ovrd=off  block_type=mux
  Relational{,1..10} (11 alike) : xbsIndex_r4/Relational  mode=a=b  op_type=Bool  en=off  latency=1  dbl_ovrd=off  block_type=relational
  ca_addr : Outport
  wires:
  [CA_code_addr_ch11] -> Mux10/3
  Mux8/1 -> Mux7/2
  Mux5/1 -> Mux4/2
  [CA_code_select_ch8] -> Relational7/1
  [CA_code_addr_ch9] -> Mux8/3
  [CA_code_select_ch7] -> Relational6/1
  Relational/1 -> Mux/1
  [CA_code_addr_ch1] -> Mux/3
  Mux9/1 -> Mux8/2
  ca_select/1 -> Relational1/2, Relational2/2, Relational3/2, Relational4/2, Relational5/2, Relational6/2, Relational7/2, Relational8/2, Relational9/2, Relational10/2, Relational/2
  Relational9/1 -> Mux9/1
  Mux3/1 -> Mux2/2
  [CA_code_select_ch4] -> Relational3/1
  [CA_code_select_ch3] -> Relational2/1
  Relational8/1 -> Mux8/1
  Relational2/1 -> Mux2/1
  [CA_code_addr_ch5] -> Mux4/3
  [CA_code_select_ch5] -> Relational4/1
  Relational10/1 -> Mux10/1
  Mux2/1 -> Mux1/2
  [CA_code_select_ch2] -> Relational1/1
  Mux4/1 -> Mux3/2
  Relational7/1 -> Mux7/1
  Relational4/1 -> Mux4/1
  [CA_code_select_ch6] -> Relational5/1
  [CA_code_addr_ch6] -> Mux5/3
  [CA_code_addr_ch3] -> Mux2/3
  [CA_code_select_ch1] -> Relational/1
  [CA_code_addr_ch4] -> Mux3/3
  Relational3/1 -> Mux3/1
  [CA_code_select_ch11] -> Relational10/1
  [CA_code_select_ch10] -> Relational9/1
  [CA_code_select_ch9] -> Relational8/1
  Relational5/1 -> Mux5/1
  Mux10/1 -> Mux9/2
  [CA_code_addr_ch10] -> Mux9/3
  Mux7/1 -> Mux6/2
  [CA_code_addr_ch12] -> Mux10/2
  Relational1/1 -> Mux1/1
  [CA_code_addr_ch8] -> Mux7/3
  [CA_code_addr_ch7] -> Mux6/3
  Mux1/1 -> Mux/2
  [CA_code_addr_ch2] -> Mux1/3
  Relational6/1 -> Mux6/1
  Mux6/1 -> Mux5/2
  Mux/1 -> ca_addr/1

== system tracker/CA_code_bank/input_router/address_router30 ==
  ca_select : Inport
  Mux{,1..10} (11 alike) : xbsIndex_r4/Mux  inputs=2  en=off  latency=1  precision=Full  arith_type=Unsigned  n_bits=16  bin_pt=14  quantization=Truncate  overflow=Wrap  dbl_ovrd=off  block_type=mux
  Relational{,1..10} (11 alike) : xbsIndex_r4/Relational  mode=a=b  op_type=Bool  en=off  latency=1  dbl_ovrd=off  block_type=relational
  ca_addr : Outport
  wires:
  [CA_code_addr_ch11] -> Mux10/3
  Mux8/1 -> Mux7/2
  Mux5/1 -> Mux4/2
  [CA_code_select_ch8] -> Relational7/1
  [CA_code_addr_ch9] -> Mux8/3
  [CA_code_select_ch7] -> Relational6/1
  Relational/1 -> Mux/1
  [CA_code_addr_ch1] -> Mux/3
  Mux9/1 -> Mux8/2
  ca_select/1 -> Relational1/2, Relational2/2, Relational3/2, Relational4/2, Relational5/2, Relational6/2, Relational7/2, Relational8/2, Relational9/2, Relational10/2, Relational/2
  Relational9/1 -> Mux9/1
  Mux3/1 -> Mux2/2
  [CA_code_select_ch4] -> Relational3/1
  [CA_code_select_ch3] -> Relational2/1
  Relational8/1 -> Mux8/1
  Relational2/1 -> Mux2/1
  [CA_code_addr_ch5] -> Mux4/3
  [CA_code_select_ch5] -> Relational4/1
  Relational10/1 -> Mux10/1
  Mux2/1 -> Mux1/2
  [CA_code_select_ch2] -> Relational1/1
  Mux4/1 -> Mux3/2
  Relational7/1 -> Mux7/1
  Relational4/1 -> Mux4/1
  [CA_code_select_ch6] -> Relational5/1
  [CA_code_addr_ch6] -> Mux5/3
  [CA_code_addr_ch3] -> Mux2/3
  [CA_code_select_ch1] -> Relational/1
  [CA_code_addr_ch4] -> Mux3/3
  Relational3/1 -> Mux3/1
  [CA_code_select_ch11] -> Relational10/1
  [CA_code_select_ch10] -> Relational9/1
  [CA_code_select_ch9] -> Relational8/1
  Relational5/1 -> Mux5/1
  Mux10/1 -> Mux9/2
  [CA_code_addr_ch10] -> Mux9/3
  Mux7/1 -> Mux6/2
  [CA_code_addr_ch12] -> Mux10/2
  Relational1/1 -> Mux1/1
  [CA_code_addr_ch8] -> Mux7/3
  [CA_code_addr_ch7] -> Mux6/3
  Mux1/1 -> Mux/2
  [CA_code_addr_ch2] -> Mux1/3
  Relational6/1 -> Mux6/1
  Mux6/1 -> Mux5/2
  Mux/1 -> ca_addr/1

== system tracker/CA_code_bank/input_router/address_router31 ==
  ca_select : Inport
  Mux{,1..10} (11 alike) : xbsIndex_r4/Mux  inputs=2  en=off  latency=1  precision=Full  arith_type=Unsigned  n_bits=16  bin_pt=14  quantization=Truncate  overflow=Wrap  dbl_ovrd=off  block_type=mux
  Relational{,1..10} (11 alike) : xbsIndex_r4/Relational  mode=a=b  op_type=Bool  en=off  latency=1  dbl_ovrd=off  block_type=relational
  ca_addr : Outport
  wires:
  Mux/1 -> ca_addr/1
  Mux6/1 -> Mux5/2
  Relational6/1 -> Mux6/1
  [CA_code_addr_ch2] -> Mux1/3
  Mux1/1 -> Mux/2
  [CA_code_addr_ch7] -> Mux6/3
  [CA_code_addr_ch8] -> Mux7/3
  Relational1/1 -> Mux1/1
  [CA_code_addr_ch12] -> Mux10/2
  Mux7/1 -> Mux6/2
  [CA_code_addr_ch10] -> Mux9/3
  Mux10/1 -> Mux9/2
  Relational5/1 -> Mux5/1
  [CA_code_select_ch9] -> Relational8/1
  [CA_code_select_ch10] -> Relational9/1
  [CA_code_select_ch11] -> Relational10/1
  Relational3/1 -> Mux3/1
  [CA_code_addr_ch4] -> Mux3/3
  [CA_code_select_ch1] -> Relational/1
  [CA_code_addr_ch3] -> Mux2/3
  [CA_code_addr_ch6] -> Mux5/3
  [CA_code_select_ch6] -> Relational5/1
  Relational4/1 -> Mux4/1
  Relational7/1 -> Mux7/1
  Mux4/1 -> Mux3/2
  [CA_code_select_ch2] -> Relational1/1
  Mux2/1 -> Mux1/2
  Relational10/1 -> Mux10/1
  [CA_code_select_ch5] -> Relational4/1
  [CA_code_addr_ch5] -> Mux4/3
  Relational2/1 -> Mux2/1
  Relational8/1 -> Mux8/1
  [CA_code_select_ch3] -> Relational2/1
  [CA_code_select_ch4] -> Relational3/1
  Mux3/1 -> Mux2/2
  Relational9/1 -> Mux9/1
  ca_select/1 -> Relational/2, Relational10/2, Relational9/2, Relational8/2, Relational7/2, Relational6/2, Relational5/2, Relational4/2, Relational3/2, Relational2/2, Relational1/2
  Mux9/1 -> Mux8/2
  [CA_code_addr_ch1] -> Mux/3
  Relational/1 -> Mux/1
  [CA_code_select_ch7] -> Relational6/1
  [CA_code_addr_ch9] -> Mux8/3
  [CA_code_select_ch8] -> Relational7/1
  Mux5/1 -> Mux4/2
  Mux8/1 -> Mux7/2
  [CA_code_addr_ch11] -> Mux10/3
